simulink model "bh_2dof_simscape_model"  (R2017a)
settings: Solver=ode45  StartTime=0.0  StopTime=20  RelTol=1e-5  EnableMultiTasking=on
PreLoadFcn:
  | bh_script_2dof_params
values from neighbouring files (symbols this model uses):
  c1 = 20    [bh_2dof_MATLAB_analysis.m]
  c2 = 50    [bh_2dof_MATLAB_analysis.m]
  c3 = 10    [bh_2dof_MATLAB_analysis.m]
libraries: fl_lib x18, nesl_utility x7
settings Model: Creator=bhorton  LastModifiedBy=bhorton
settings OptimizationCC: LifeSpan=inf
settings DebuggingCC: SFUnexpectedBacktrackingDiag=warning  SFNoUnconditionalDefaultTransitionDiag=warning  SFExecutionAtInitializationDiag=none
settings GRTTargetCC: TargetLangStandard=C89/C90 (ANSI)  GeneratePreprocessorConditionals=Disable all
settings ConfigComp: CovMetricSettings=dw  CovHtmlReporting=on  CovSaveCumulativeToWorkspaceVar=on  CovSaveSingleToWorkspaceVar=on  CovExternalEMLEnable=off

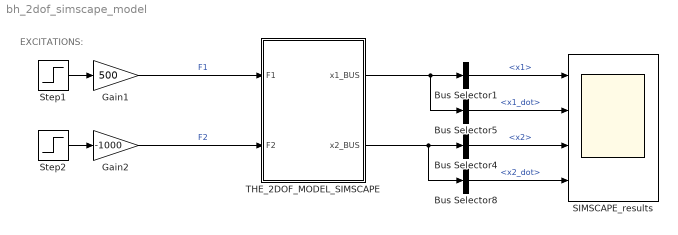
== system bh_2dof_simscape_model ==
  note: EXCITATIONS:
  Bus Selector1 : BusSelector  OutputSignals=x1
  Bus Selector4 : BusSelector  OutputSignals=x2
  Bus Selector5 : BusSelector  OutputSignals=x1_dot
  Bus Selector8 : BusSelector  OutputSignals=x2_dot
  Gain1 : Gain  Gain=500
  Gain2 : Gain  Gain=-1000
  SIMSCAPE_results : Scope  NumInputPorts=4
  Step1 : Step  Time=5  SampleTime=0
  Step2 : Step  Time=10  SampleTime=0
  THE_2DOF_MODEL_SIMSCAPE : Subsystem
  wires:
  Step1/1 -> Gain1/1
  Gain1/1 -> THE_2DOF_MODEL_SIMSCAPE/1(F1)  "F1"
  Step2/1 -> Gain2/1
  Gain2/1 -> THE_2DOF_MODEL_SIMSCAPE/2(F2)  "F2"
  Bus Selector1/1 -> SIMSCAPE_results/1  "<x1>"
  Bus Selector4/1 -> SIMSCAPE_results/3  "<x2>"
  Bus Selector5/1 -> SIMSCAPE_results/2  "<x1_dot>"
  Bus Selector8/1 -> SIMSCAPE_results/4  "<x2_dot>"
  THE_2DOF_MODEL_SIMSCAPE/2(x2_BUS) -> Bus Selector8/1, Bus Selector4/1
  THE_2DOF_MODEL_SIMSCAPE/1(x1_BUS) -> Bus Selector5/1, Bus Selector1/1

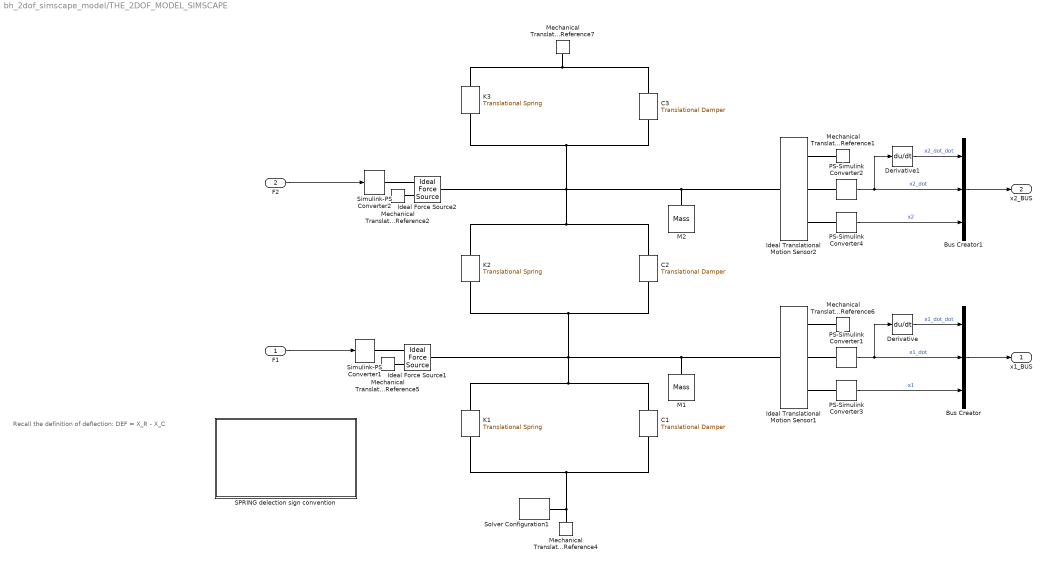
== system bh_2dof_simscape_model/THE_2DOF_MODEL_SIMSCAPE ==
  note: Recall the definition of deflection:
      |
      |          DEF = X_R - X_C
  F1 : Inport
  F2 : Inport  Port=2
  Bus Creator : BusCreator  Inputs=3
  Bus Creator1 : BusCreator  Inputs=3
  C1 : fl_lib/Mechanical/Translational Elements/Translational Damper  D=c1 N/(m/s)  v_specify=off  v_priority=None  v=0 m/s  v_nominal_specify=off  v_nominal_unit=m/s  v_nominal_value=1  f_specify=off  f_priority=None  f=0 N  f_nominal_specify=off  f_nominal_unit=N  f_nominal_value=1
      settings: AttributesFormatString=C= %<D>
  C2 : fl_lib/Mechanical/Translational Elements/Translational Damper  D=c2 N/(m/s)  v_specify=off  v_priority=None  v=0 m/s  v_nominal_specify=off  v_nominal_unit=m/s  v_nominal_value=1  f_specify=off  f_priority=None  f=0 N  f_nominal_specify=off  f_nominal_unit=N  f_nominal_value=1
      settings: AttributesFormatString=C= %<D>
  C3 : fl_lib/Mechanical/Translational Elements/Translational Damper  D=c3 N/(m/s)  v_specify=off  v_priority=None  v=0 m/s  v_nominal_specify=off  v_nominal_unit=m/s  v_nominal_value=1  f_specify=off  f_priority=None  f=0 N  f_nominal_specify=off  f_nominal_unit=N  f_nominal_value=1
      settings: AttributesFormatString=C= %<D>
  Derivative : Derivative
  Derivative1 : Derivative
  Ideal Force Source1 : fl_lib/Mechanical/Mechanical Sources/Ideal Force Source
  Ideal Force Source2 : fl_lib/Mechanical/Mechanical Sources/Ideal Force Source
  Ideal Translational Motion Sensor1 : fl_lib/Mechanical/Mechanical Sensors/Ideal Translational Motion Sensor  offset=def_k1.xC m
      settings: AttributesFormatString=INITIAL_POS= %<offset>
  Ideal Translational Motion Sensor2 : fl_lib/Mechanical/Mechanical Sensors/Ideal Translational Motion Sensor  offset=def_k2.xC m
      settings: AttributesFormatString=INITIAL_POS= %<offset>
  K1 : fl_lib/Mechanical/Translational Elements/Translational Spring  spr_rate=k1 N/m  v_specify=off  v_priority=High  v=0 m/s  v_nominal_specify=off  v_nominal_unit=m/s  v_nominal_value=1  f_specify=off  f_priority=None  f=0 N  f_nominal_specify=off  f_nominal_unit=N  f_nominal_value=1  x_specify=on  x_priority=High  x=def_k1.x_def m  x_nominal_specify=off  x_nominal_unit=m  x_nominal_value=1
      settings: AttributesFormatString=|
      | K= %<spr_rate>
      | X_DEF= %<x>
  K2 : fl_lib/Mechanical/Translational Elements/Translational Spring  spr_rate=k2 N/m  v_specify=off  v_priority=High  v=0 m/s  v_nominal_specify=off  v_nominal_unit=m/s  v_nominal_value=1  f_specify=off  f_priority=None  f=0 N  f_nominal_specify=off  f_nominal_unit=N  f_nominal_value=1  x_specify=on  x_priority=High  x=def_k2.x_def m  x_nominal_specify=off  x_nominal_unit=m  x_nominal_value=1
      settings: AttributesFormatString=|
      | K= %<spr_rate>
      | X_DEF= %<x>
  K3 : fl_lib/Mechanical/Translational Elements/Translational Spring  spr_rate=k3 N/m  v_specify=off  v_priority=High  v=0 m/s  v_nominal_specify=off  v_nominal_unit=m/s  v_nominal_value=1  f_specify=off  f_priority=None  f=0 N  f_nominal_specify=off  f_nominal_unit=N  f_nominal_value=1  x_specify=on  x_priority=High  x=def_k3.x_def m  x_nominal_specify=off  x_nominal_unit=m  x_nominal_value=1
      settings: AttributesFormatString=|
      | K= %<spr_rate>
      | X_DEF= %<x>
  M1 : fl_lib/Mechanical/Translational Elements/Mass  mass=m1 kg  v_specify=on  v_priority=High  v=def_k1.vC m/s  v_nominal_specify=off  v_nominal_unit=m/s  v_nominal_value=1  f_specify=off  f_priority=None  f=0 N  f_nominal_specify=off  f_nominal_unit=N  f_nominal_value=1
      settings: AttributesFormatString=|
      | m= %<mass>
      | v = %<v>
  M2 : fl_lib/Mechanical/Translational Elements/Mass  mass=m2 kg  v_specify=on  v_priority=High  v=def_k2.vC m/s  v_nominal_specify=off  v_nominal_unit=m/s  v_nominal_value=1  f_specify=off  f_priority=None  f=0 N  f_nominal_specify=off  f_nominal_unit=N  f_nominal_value=1
      settings: AttributesFormatString=|
      | m= %<mass>
      | v = %<v>
  Mechanical Translational Reference{1..2,4..7} (6 alike) : fl_lib/Mechanical/Translational Elements/Mechanical Translational Reference
  PS-Simulink Converter1 : nesl_utility/PS-Simulink Converter  PhysicalDomain=network_engine_domain  SubClassName=ps_output  LeftPortType=input  RightPortType=output  PseudoPeriodic=off  Frequencies=[]  Unit=m/s  AffineConversion=off
  PS-Simulink Converter2 : nesl_utility/PS-Simulink Converter  PhysicalDomain=network_engine_domain  SubClassName=ps_output  LeftPortType=input  RightPortType=output  PseudoPeriodic=off  Frequencies=[]  Unit=m/s  AffineConversion=off
  PS-Simulink Converter3 : nesl_utility/PS-Simulink Converter  PhysicalDomain=network_engine_domain  SubClassName=ps_output  LeftPortType=input  RightPortType=output  PseudoPeriodic=off  Frequencies=[]  Unit=m  AffineConversion=off
  PS-Simulink Converter4 : nesl_utility/PS-Simulink Converter  PhysicalDomain=network_engine_domain  SubClassName=ps_output  LeftPortType=input  RightPortType=output  PseudoPeriodic=off  Frequencies=[]  Unit=m  AffineConversion=off
  SPRING delection sign convention : Subsystem
  Simulink-PS Converter1 : nesl_utility/Simulink-PS Converter  PhysicalDomain=network_engine_domain  SubClassName=ps_input  LeftPortType=input  RightPortType=output  PseudoPeriodic=off  Frequencies=[]  NoiseDistribution=none  NoiseParameters=[]  Unit=N  AffineConversion=off  FilteringAndDerivatives=zero  SimscapeFilterOrder=1  InputFilterTimeConstant=0.001  UdotUserProvided=1
  Simulink-PS Converter2 : nesl_utility/Simulink-PS Converter  PhysicalDomain=network_engine_domain  SubClassName=ps_input  LeftPortType=input  RightPortType=output  PseudoPeriodic=off  Frequencies=[]  NoiseDistribution=none  NoiseParameters=[]  Unit=N  AffineConversion=off  FilteringAndDerivatives=zero  SimscapeFilterOrder=1  InputFilterTimeConstant=0.001  UdotUserProvided=1
  Solver Configuration1 : nesl_utility/Solver Configuration  PhysicalDomain=network_engine_domain  SubClassName=solver  LeftPortType=input  RightPortType=generic  Accelerate=off  Tones=[]  Harmonics=[]  SimulateNoise=off  Profile=off  UseLocalSampling=off  EnableSwitchedLinearOptims=on  FrequencyDomain=off  UseCCode=off  RelTol=0.001  AbsTol=1e-06  MinStep=1e-09  ToWorkspace=off  RevertToSquareIcSolve=off  NumHomotopyIterations=100  PhasorMode=off  PhasorModeNumHarmonics=1  OverrideAbsTol=off  DoDC=off  ResidualTolerance=1e-09  UseLocalSolver=off  LocalSolverChoice=NE_BACKWARD_EULER_ADVANCER  LocalSolverSampleTime=0.001  DoFixedCost=off  MaxNonlinIter=3  MaxModeIter=2  LinearAlgebra=Sparse  DelaysMemoryBudget=1024  AutomaticFiltering=on  FilteringTimeConstant=0.001
  x1_BUS : Outport
  x2_BUS : Outport  Port=2
  wires:
  F1/1 -> Simulink-PS Converter1/1
  PS-Simulink Converter1/1 -> Bus Creator/2, Derivative/1  "x1_dot"
  Derivative/1 -> Bus Creator/1  "x1_dot_dot"
  PS-Simulink Converter3/1 -> Bus Creator/3  "x1"
  PS-Simulink Converter2/1 -> Bus Creator1/2, Derivative1/1  "x2_dot"
  Derivative1/1 -> Bus Creator1/1  "x2_dot_dot"
  PS-Simulink Converter4/1 -> Bus Creator1/3  "x2"
  F2/1 -> Simulink-PS Converter2/1
  Bus Creator/1 -> x1_BUS/1
  Bus Creator1/1 -> x2_BUS/1
  connections:
  Mechanical Translational Reference4/LConn1 -- Solver Configuration1/RConn1 -- K1/LConn1 -- C1/LConn1
  C1/RConn1 -- K1/RConn1 -- Ideal Translational Motion Sensor1/LConn1 -- M1/LConn1 -- Ideal Force Source1/LConn1 -- C2/LConn1 -- K2/LConn1
  Ideal Force Source2/LConn1 -- M2/LConn1 -- Ideal Translational Motion Sensor2/LConn1 -- K2/RConn1 -- C2/RConn1 -- C3/LConn1 -- K3/LConn1
  Mechanical Translational Reference7/LConn1 -- C3/RConn1 -- K3/RConn1
  Simulink-PS Converter2/RConn1 -- Ideal Force Source2/RConn1
  Mechanical Translational Reference2/LConn1 -- Ideal Force Source2/RConn2
  PS-Simulink Converter2/LConn1 -- Ideal Translational Motion Sensor2/RConn2
  Mechanical Translational Reference1/LConn1 -- Ideal Translational Motion Sensor2/RConn1
  Ideal Translational Motion Sensor2/RConn3 -- PS-Simulink Converter4/LConn1
  Mechanical Translational Reference6/LConn1 -- Ideal Translational Motion Sensor1/RConn1
  PS-Simulink Converter1/LConn1 -- Ideal Translational Motion Sensor1/RConn2
  Mechanical Translational Reference5/LConn1 -- Ideal Force Source1/RConn2
  Ideal Translational Motion Sensor1/RConn3 -- PS-Simulink Converter3/LConn1
  Simulink-PS Converter1/RConn1 -- Ideal Force Source1/RConn1

== system bh_2dof_simscape_model/THE_2DOF_MODEL_SIMSCAPE/SPRING delection sign convention ==
  note: deflection is NEGATIVE (-)
  note: deflection is POSITIVE (+)
  note: Recall the definition of deflection:
      |
      |          DEF = X_R - X_C
